simulink model "EX2_zadanie1"  (R2023b)
settings: Solver=FixedStepDiscrete  StartTime=0.0  StopTime=0  RelTol=1e-3
libraries: CPOiS_SourcesSinks x7, CPOiS_HistogramOperations x3
settings Model: Creator=alyskawa  LastModifiedBy=alyskawa

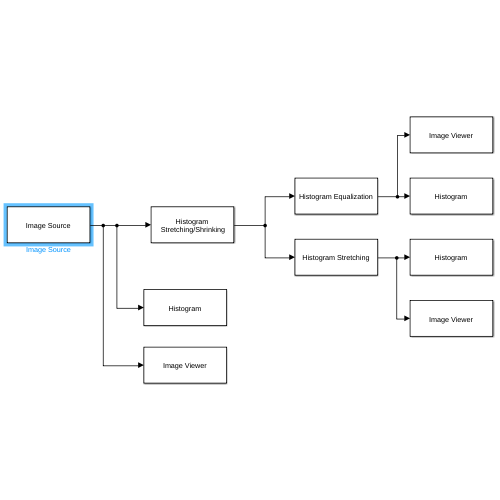
[thumbnail: Simulink's stored preview of the top-level diagram]
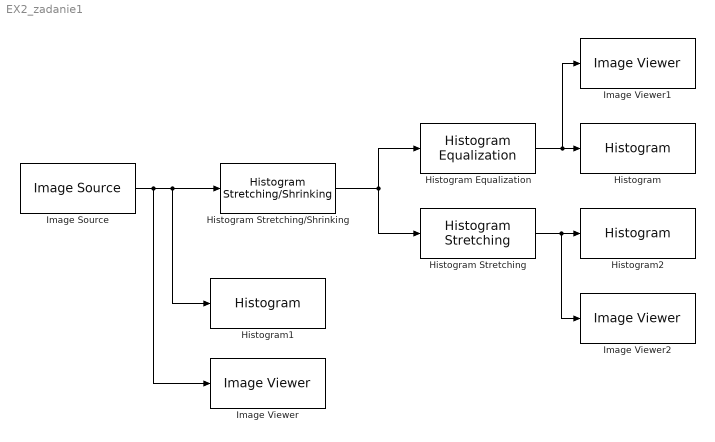
== system EX2_zadanie1 ==
  Histogram : CPOiS_SourcesSinks/Histogram
      settings: SourceProductName=CPOiS - Digital image and signal processing
  Histogram Stretching/Shrinking : CPOiS_HistogramOperations/Histogram Stretching//Shrinking  minimum=0  maximum=255
      settings: SourceProductName=CPOiS - Digital image and signal processing
  Histogram Equalization : CPOiS_HistogramOperations/Histogram Equalization
      settings: SourceProductName=CPOiS - Digital image and signal processing
  Histogram Stretching : CPOiS_HistogramOperations/Histogram Stretching
      settings: SourceProductName=CPOiS - Digital image and signal processing
  Histogram1 : CPOiS_SourcesSinks/Histogram
      settings: SourceProductName=CPOiS - Digital image and signal processing
  Histogram2 : CPOiS_SourcesSinks/Histogram
      settings: SourceProductName=CPOiS - Digital image and signal processing
  Image Source : CPOiS_SourcesSinks/Image Source  FileSelection=airport.png
      settings: SourceProductName=CPOiS - Digital image and signal processing
  Image Viewer : CPOiS_SourcesSinks/Image Viewer
      settings: SourceProductName=CPOiS - Digital image and signal processing
  Image Viewer1 : CPOiS_SourcesSinks/Image Viewer
      settings: SourceProductName=CPOiS - Digital image and signal processing
  Image Viewer2 : CPOiS_SourcesSinks/Image Viewer
      settings: SourceProductName=CPOiS - Digital image and signal processing
  wires:
  Image Source/1 -> Histogram Stretching/Shrinking/1, Histogram1/1, Image Viewer/1
  Histogram Stretching/Shrinking/1 -> Histogram Stretching/1, Histogram Equalization/1
  Histogram Stretching/1 -> Image Viewer2/1, Histogram2/1
  Histogram Equalization/1 -> Image Viewer1/1, Histogram/1
